simulink model "BLDC"  (R2023a)
settings: Solver=VariableStepAuto  StartTime=0.0  StopTime=10.0  RelTol=1e-3
libraries: spsControlledVoltageSourceLib x1, spsPermanentMagnetSynchronousMachineLib x1, spsUniversalBridgeLib x1, spsVoltageMeasurementLib x1
settings Model: Creator=Hp  LastModifiedBy=Hp

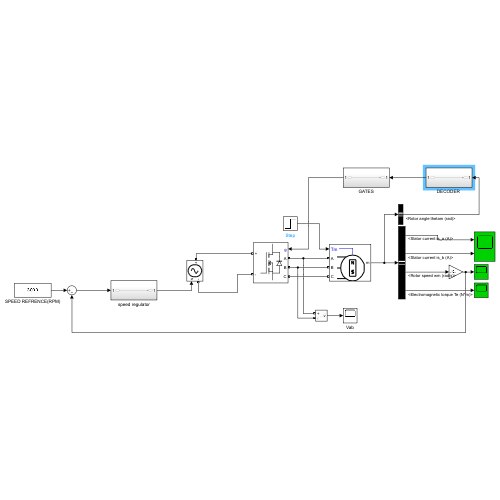
[thumbnail: Simulink's stored preview of the top-level diagram]
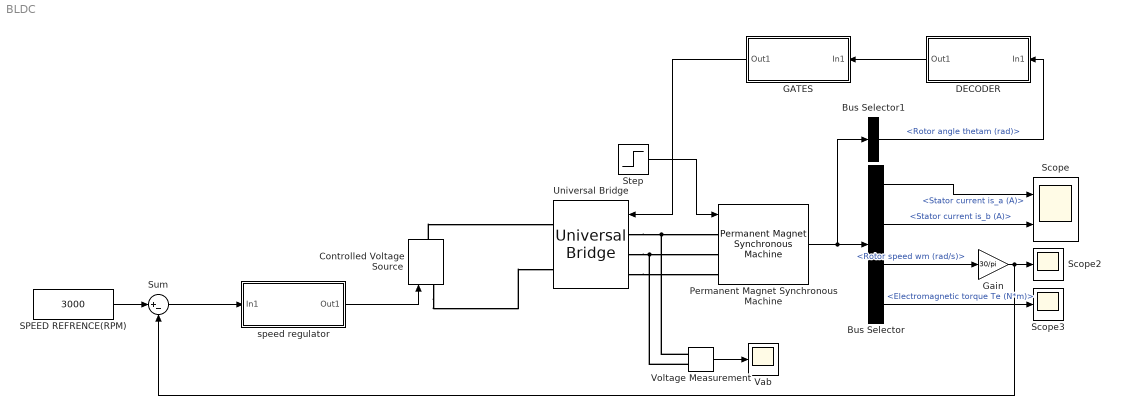
== system BLDC ==
  Bus Selector : BusSelector  OutputSignals=Stator current is_a (A),Stator current is_b (A),Rotor speed wm (rad/s),Electromagnetic torque Te (N*m)
  Bus Selector1 : BusSelector  OutputSignals=Rotor angle thetam (rad)
  Controlled Voltage Source : spsControlledVoltageSourceLib/Controlled Voltage Source  Initialize=on  Source_Type=AC  Amplitude=0  Phase=0  Frequency=0  Measurements=None
  "DECODER " : Subsystem
  GATES : Subsystem
  Gain : Gain  Gain=30/pi
  Permanent Magnet Synchronous Machine : spsPermanentMagnetSynchronousMachineLib/Permanent Magnet Synchronous Machine  NbPhases=3  FluxDistribution=Trapezoidal  RotorType=Round  MechanicalLoad=Torque Tm  PresetModel=No  ShowDetailedParameters=on  MeasurementBus=off  Resistance=0.0485  Inductance=8.5e-3  dqInductances=[8.5e-3,8.5e-3]  La=0.000395  MachineConstant=Flux linkage established by magnets (V.s)  Flux=0.1194  VoltageCst=100.0283  TorqueCst=0.9552  Flat=120  Mechanical=[0.0027 0.0004924 4 0]  PolePairs=4  InitialConditions=[0,0, 0,0]  InitialConditions5ph=[0 0 0 0 0 0]  RefAngle=90 degrees behind phase A axis (modified Park)  IterativeDiscreteModel=Trapezoidal non iterative  TsBlock=-1  TsPowergui=0
  SPEED REFRENCE(RPM) : Constant  Value=3000
  Scope : Scope  NumInputPorts=2
  Scope2 : Scope
  Scope3 : Scope
  Step : Step  SampleTime=0
  Sum : Sum  Inputs=|+-
  Universal Bridge : spsUniversalBridgeLib/Universal Bridge  Arms=3  SnubberResistance=1e5  SnubberCapacitance=inf  Device=MOSFET / Diodes  Ron=1e-3  Lon=0  ForwardVoltages="[  0  0  ]"  ForwardVoltage=0  GTOparameters=[ 10e-6 , 20e-6 ]  IGBTparameters=[ 1e-6 , 2e-6 ]  Measurements=None  Measurements_2=None  converterType=Rectifier
  Vab : Scope
  Voltage Measurement : spsVoltageMeasurementLib/Voltage Measurement  PhasorSimulation=off  OutputType=Complex  PSBequivalent=0
  speed regulator : Subsystem
  wires:
  speed regulator/1(Out1) -> Controlled Voltage Source/1
  Sum/1 -> speed regulator/1(In1)
  SPEED REFRENCE(RPM)/1 -> Sum/1
  "DECODER "/1(Out1) -> GATES/1(In1)
  GATES/1(Out1) -> Universal Bridge/1
  Step/1 -> Permanent Magnet Synchronous Machine/1
  Permanent Magnet Synchronous Machine/1 -> Bus Selector1/1, Bus Selector/1
  Bus Selector1/1 -> "DECODER "/1(In1)  "<Rotor angle thetam (rad)>"
  Bus Selector/1 -> Scope/1  "<Stator current is_a (A)>"
  Bus Selector/3 -> Gain/1  "<Rotor speed wm (rad/s)>"
  Bus Selector/4 -> Scope3/1  "<Electromagnetic torque Te (N*m)>"
  Gain/1 -> Sum/2, Scope2/1
  Bus Selector/2 -> Scope/2  "<Stator current is_b (A)>"
  Voltage Measurement/1 -> Vab/1
  connections:
  Universal Bridge/LConn1 -- Voltage Measurement/LConn1 -- Permanent Magnet Synchronous Machine/LConn1
  Universal Bridge/LConn2 -- Voltage Measurement/LConn2 -- Permanent Magnet Synchronous Machine/LConn2
  Universal Bridge/LConn3 -- Permanent Magnet Synchronous Machine/LConn3
  Controlled Voltage Source/RConn1 -- Universal Bridge/RConn1
  Controlled Voltage Source/LConn1 -- Universal Bridge/RConn2

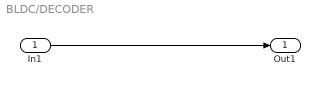
== system BLDC/DECODER  ==
  In1 : Inport
  Out1 : Outport
  wires:
  In1/1 -> Out1/1

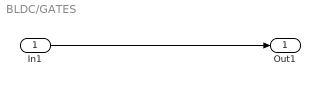
== system BLDC/GATES ==
  In1 : Inport
  Out1 : Outport
  wires:
  In1/1 -> Out1/1

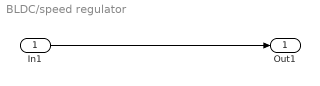
== system BLDC/speed regulator ==
  In1 : Inport
  Out1 : Outport
  wires:
  In1/1 -> Out1/1
